simulink model "openLoopExperiments"  (R2020b)
settings: Solver=VariableStepAuto  StartTime=0.0  StopTime=300  MaxStep=0.01  RelTol=1e-3
values from neighbouring files (symbols this model uses):
  k = 10    [params.m]
  m = 1    [params.m]
undefined symbols (not defined in the file or in its folder): c
settings Model: Creator=kaijunge  LastModifiedBy=kaijunge
settings ExplorerConfigSet: SimMechanicsOpenEditorOnUpdate=off

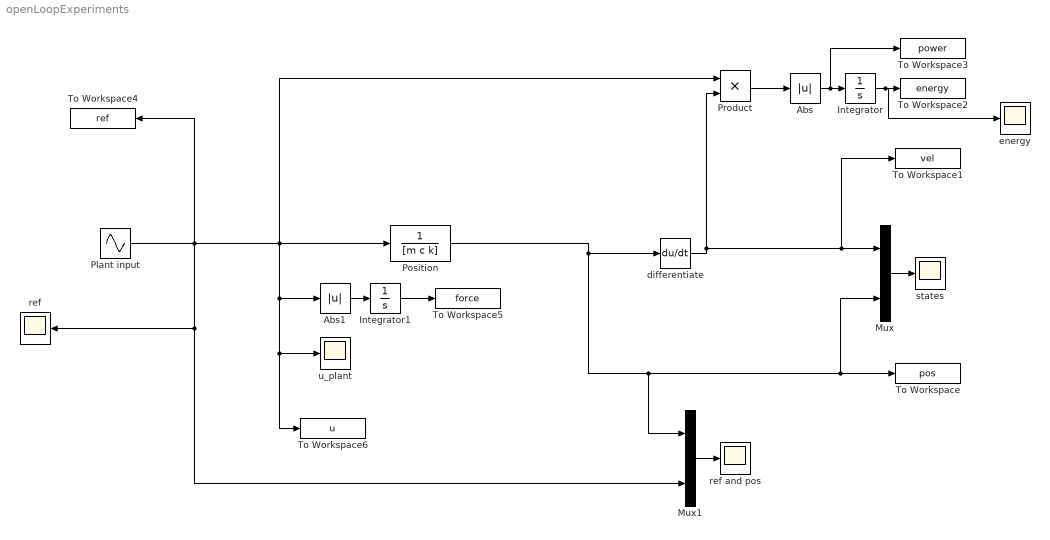
== system openLoopExperiments ==
  Abs : Abs
  Abs1 : Abs
  Integrator : Integrator
  Integrator1 : Integrator
  Mux : Mux  Inputs=2
  Mux1 : Mux  Inputs=2
  Plant input : Sin  Frequency=0.9  SampleTime=0
  Position : TransferFcn  Denominator=[m c k]
  Product : Product
  To Workspace : ToWorkspace  VariableName=pos  SaveFormat=Timeseries  SampleTime=-1
  To Workspace1 : ToWorkspace  VariableName=vel  SaveFormat=Timeseries  SampleTime=-1
  To Workspace2 : ToWorkspace  VariableName=energy  SaveFormat=Timeseries  SampleTime=-1
  To Workspace3 : ToWorkspace  VariableName=power  SaveFormat=Timeseries  SampleTime=-1
  To Workspace4 : ToWorkspace  VariableName=ref  SaveFormat=Timeseries  SampleTime=-1
  To Workspace5 : ToWorkspace  VariableName=force  SaveFormat=Timeseries  SampleTime=-1
  To Workspace6 : ToWorkspace  VariableName=u  SaveFormat=Timeseries  SampleTime=-1
  differentiate : Derivative
  energy : Scope
  ref : Scope
  ref and pos : Scope
  states : Scope
  u_plant : Scope
  wires:
  Abs/1 -> To Workspace3/1, Integrator/1
  Integrator1/1 -> To Workspace5/1
  Plant input/1 -> ref/1, Mux1/2, u_plant/1, To Workspace6/1, Abs1/1, Position/1, Product/1, To Workspace4/1
  Integrator/1 -> To Workspace2/1, energy/1
  Product/1 -> Abs/1
  differentiate/1 -> Product/2, To Workspace1/1, Mux/1
  Mux/1 -> states/1
  Abs1/1 -> Integrator1/1
  Position/1 -> differentiate/1, Mux1/1, Mux/2, To Workspace/1
  Mux1/1 -> ref and pos/1
